simulink model "sys_ctrl_obs_luenberger_full_lineal"  (Simulink 8.6)
settings: Solver=ode45  StartTime=0.0  StopTime=Tt  RelTol=1e-3
undefined symbols (not defined in the file): Ad, Bd, Cd, Dd, K, Knoise, L, r, Ts, x_0
settings Model: Creator=pdoren  LastModifiedBy=pdoren
settings SolverCC: ZeroCrossAlgorithm=Adaptive
settings DataIOCC: SaveFormat=StructureWithTime  SignalLoggingSaveFormat=Dataset
settings OptimizationCC: ExpressionDepthLimit=128
settings DebuggingCC: UnderspecifiedInitializationDetection=Simplified  MergeDetectMultiDrivingBlocksExec=error  SolverPrmCheckMsg=none  FcnCallInpInsideContextMsg=EnableAllAsWarning  StateNameClashWarn=none
settings HardwareCC: ProdBitPerPointer=64  ProdLargestAtomicFloat=Float  ProdIntDivRoundTo=Zero  ProdEndianess=LittleEndian  ProdHWDeviceType=Specified
settings GRTTargetCC: GeneratePreprocessorConditionals=Use local settings
settings ConfigComp: CovModelRefEnable=off

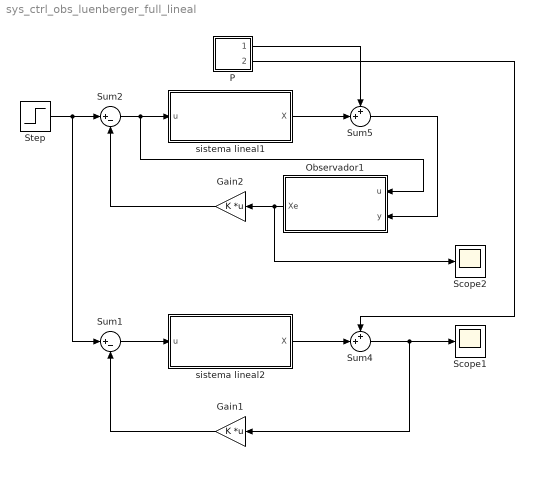
== system sys_ctrl_obs_luenberger_full_lineal ==
  Gain1 : Gain  Gain=K  Multiplication=Matrix(K*u)
  Gain2 : Gain  Gain=K  Multiplication=Matrix(K*u)
  Observador1 : Subsystem
  P : Subsystem
  Scope1 : Scope
  Scope2 : Scope
  Step : Step  After=r  SampleTime=0
  Sum1 : Sum  Inputs=|+-
  Sum2 : Sum  Inputs=|+-
  Sum4 : Sum  Inputs=++|
  Sum5 : Sum  Inputs=++|
  sistema lineal1 : Subsystem
  sistema lineal2 : Subsystem
  wires:
  Sum2/1 -> Observador1/1(u), sistema lineal1/1(u)
  Gain2/1 -> Sum2/2
  sistema lineal1/1(X) -> Sum5/2
  Step/1 -> Sum1/1, Sum2/1
  Sum1/1 -> sistema lineal2/1(u)
  Gain1/1 -> Sum1/2
  sistema lineal2/1(X) -> Sum4/2
  Sum4/1 -> Gain1/1, Scope1/1
  P/2(Noise4) -> Sum4/1
  P/1(Noise2) -> Sum5/1
  Observador1/1(Xe) -> Gain2/1, Scope2/1
  Sum5/1 -> Observador1/2(y)

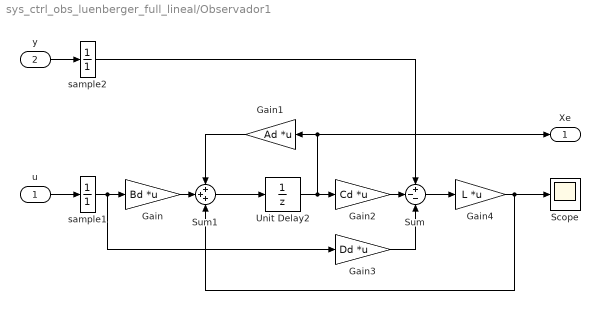
== system sys_ctrl_obs_luenberger_full_lineal/Observador1 ==
  u : Inport
  y : Inport  Port=2
  Gain : Gain  Gain=Bd  Multiplication=Matrix(K*u)
  Gain1 : Gain  Gain=Ad  Multiplication=Matrix(K*u)
  Gain2 : Gain  Gain=Cd  Multiplication=Matrix(K*u)
  Gain3 : Gain  Gain=Dd  Multiplication=Matrix(K*u)
  Gain4 : Gain  Gain=L  Multiplication=Matrix(K*u)
  Scope : Scope
  Sum : Sum  Inputs=+--
  Sum1 : Sum  Inputs=+++
  Unit Delay2 : UnitDelay  SampleTime=Ts
  sample1 : DiscreteTransferFcn  Denominator=[1]  SampleTime=Ts
  sample2 : DiscreteTransferFcn  Denominator=[1]  SampleTime=Ts
  Xe : Outport
  wires:
  Unit Delay2/1 -> Gain2/1, Xe/1, Gain1/1
  u/1 -> sample1/1
  sample1/1 -> Gain/1, Gain3/1
  Sum/1 -> Gain4/1
  y/1 -> sample2/1
  sample2/1 -> Sum/1
  Gain3/1 -> Sum/3
  Gain2/1 -> Sum/2
  Gain/1 -> Sum1/2
  Gain4/1 -> Sum1/3, Scope/1
  Gain1/1 -> Sum1/1
  Sum1/1 -> Unit Delay2/1

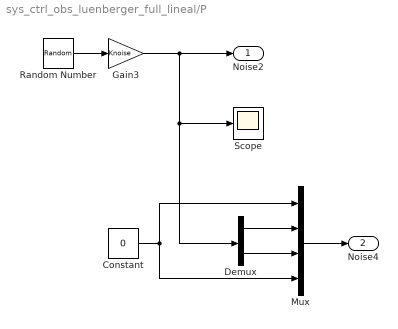
== system sys_ctrl_obs_luenberger_full_lineal/P ==
  Constant : Constant  Value=0
  Demux : Demux  Outputs=2
  Gain3 : Gain  Gain=Knoise
  Mux : Mux
  Random Number : RandomNumber  SampleTime=Ts
  Scope : Scope
  Noise2 : Outport
  Noise4 : Outport  Port=2
  wires:
  Random Number/1 -> Gain3/1
  Gain3/1 -> Noise2/1, Demux/1, Scope/1
  Mux/1 -> Noise4/1
  Demux/1 -> Mux/2
  Demux/2 -> Mux/3
  Constant/1 -> Mux/4, Mux/1

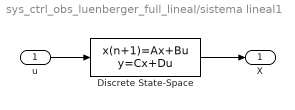
== system sys_ctrl_obs_luenberger_full_lineal/sistema lineal1 ==
  u : Inport
  Discrete State-Space : DiscreteStateSpace  A=Ad  B=Bd  C=Cd  D=Dd  X0=x_0  SampleTime=Ts
  X : Outport
  wires:
  u/1 -> Discrete State-Space/1
  Discrete State-Space/1 -> X/1

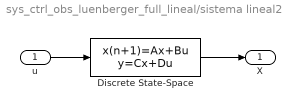
== system sys_ctrl_obs_luenberger_full_lineal/sistema lineal2 ==
  u : Inport
  Discrete State-Space : DiscreteStateSpace  A=Ad  B=Bd  C=eye(4)  D=zeros(4,1)  X0=x_0  SampleTime=Ts
  X : Outport
  wires:
  u/1 -> Discrete State-Space/1
  Discrete State-Space/1 -> X/1
